simulink model "Simulink1"  (R2018b)
settings: Solver=VariableStepAuto  StartTime=0.0  StopTime=20  RelTol=1e-3
libraries: Solver_SF x1
settings Model: Creator=孙重豪  LastModifiedBy=孙重豪

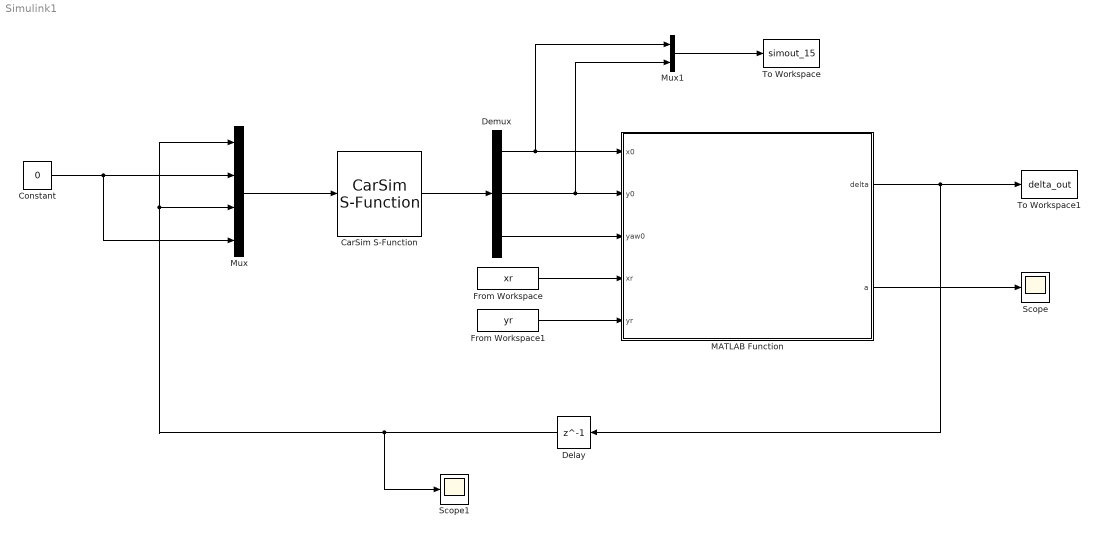
== system Simulink1 ==
  CarSim S-Function : Solver_SF/CarSim S-Function  Priority=1  SIMFILE=simfile.sim
  Constant : Constant  Value=0
  Delay : Delay  DelayLength=1  InitialCondition=0
  Demux : Demux  Outputs=3
  From Workspace : FromWorkspace  VariableName=xr  SampleTime=0
  From Workspace1 : FromWorkspace  VariableName=yr  SampleTime=0
  MATLAB Function : MATLAB Function  TreatAsAtomicUnit=on
  Mux : Mux
  Mux1 : Mux  Inputs=2
  Scope : Scope
  Scope1 : Scope
  To Workspace : ToWorkspace  VariableName=simout_15  SaveFormat=Timeseries  SampleTime=-1
      settings: Decimation=2
  To Workspace1 : ToWorkspace  VariableName=delta_out  SaveFormat=Timeseries  SampleTime=-1
  wires:
  CarSim S-Function/1 -> Demux/1
  Mux/1 -> CarSim S-Function/1
  Demux/2 -> Mux1/2, MATLAB Function/2(y0)
  Demux/1 -> Mux1/1, MATLAB Function/1(x0)
  Demux/3 -> MATLAB Function/3(yaw0)
  MATLAB Function/1(delta) -> To Workspace1/1, Delay/1
  Constant/1 -> Mux/4, Mux/2
  Delay/1 -> Scope1/1, Mux/3, Mux/1
  From Workspace/1 -> MATLAB Function/4(xr)
  From Workspace1/1 -> MATLAB Function/5(yr)
  MATLAB Function/2(a) -> Scope/1
  Mux1/1 -> To Workspace/1

== matlab function Simulink1/MATLAB Function ==
  data: x0 input; delta output; y0 input; yaw0 input; xr input; yr input; a output
function [delta, a]= fcn(x0,y0,yaw0,xr,yr)
l = 2.5;
L = 2.91;
dis = sqrt((xr-x0).^2+(yr-y0).^2);
i = find(dis==min(dis));
if(2000-i)>25
    j = l*10 + i;  % 预瞄距离    
else
    j = 2000;
end


x_pre = xr(j);
y_pre = yr(j);



a = atan((y_pre(1)-y0) / (x_pre(1)-x0)) - yaw0 * pi / 180;
delta = 1 * atan(2 * L * sin(a) / l) * 180 / pi;
